simulink model "Quadrotor_Observer"  (Simulink 7.7)
settings: Solver=ode45  StartTime=0.0  StopTime=2  RelTol=1e-3
undefined symbols (not defined in the file or in its folder): quad
settings Model: Creator=Alexey  LastModifiedBy=Alexey

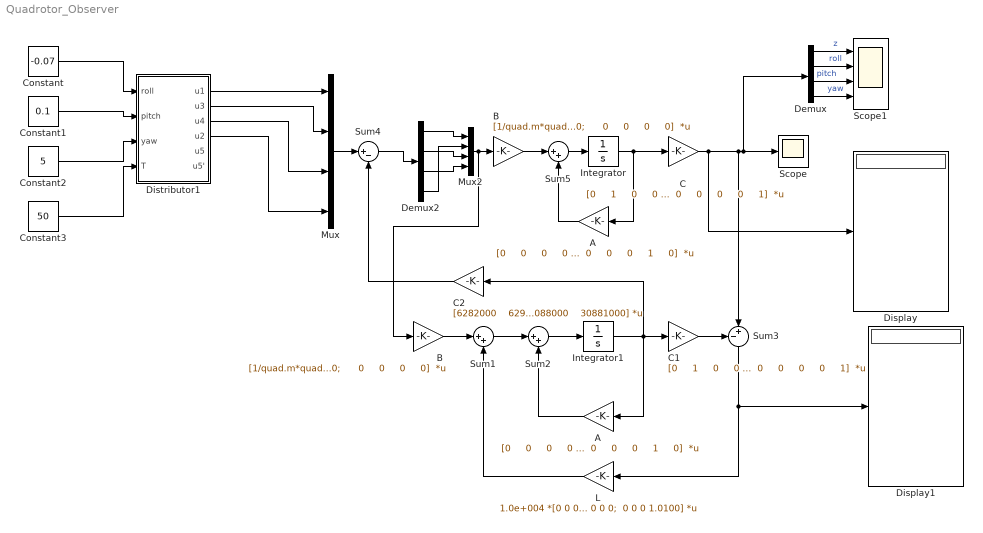
== system Quadrotor_Observer ==
  A : Gain  Gain=|  Multiplication=Matrix(K*u)
      | [0     0     0     0     0     0     0     0;
      |      1     0     0     0     0     0     0     0;
      |      0     0     0     0     0     0     0     0;
      |      0     0     1     0     0     0     0     0;
      |      0     0     0     0     0     0     0     0;
      |      0     0     0     0     1     0     0     0;
      |      0     0     0     0     0     0     0     0;
      |      0     0     0     0     0     0     1     0]
  "A " : Gain  Gain=|  Multiplication=Matrix(K*u)
      | [0     0     0     0     0     0     0     0;
      |      1     0     0     0     0     0     0     0;
      |      0     0     0     0     0     0     0     0;
      |      0     0     1     0     0     0     0     0;
      |      0     0     0     0     0     0     0     0;
      |      0     0     0     0     1     0     0     0;
      |      0     0     0     0     0     0     0     0;
      |      0     0     0     0     0     0     1     0]
  B : Gain  Gain=|  Multiplication=Matrix(K*u)
      | [1/quad.m*quad.b     0     0     0;
      |      0     0     0     0;
      |      0     0     1/quad.Ixx*quad.b*quad.l     0;
      |      0     0     0     0;
      |      0     0     0     1/quad.Iyy*quad.b*quad.l;
      |      0     0     0     0;
      |      0     1/quad.Izz*quad.k     0     0;
      |      0     0     0     0]
  "B " : Gain  Gain=|  Multiplication=Matrix(K*u)
      | [1/quad.m*quad.b     0     0     0;
      |      0     0     0     0;
      |      0     0     1/quad.Ixx*quad.b*quad.l     0;
      |      0     0     0     0;
      |      0     0     0     1/quad.Iyy*quad.b*quad.l;
      |      0     0     0     0;
      |      0     1/quad.Izz*quad.k*quad.r     0     0;
      |      0     0     0     0]
  C : Gain  Gain=|  Multiplication=Matrix(K*u)
      | [0     1     0     0     0     0     0     0;
      |      0     0     0     1     0     0     0     0;
      |      0     0     0     0     0     1     0     0;
      |      0     0     0     0     0     0     0     1]
  C1 : Gain  Gain=|  Multiplication=Matrix(K*u)
      | [0     1     0     0     0     0     0     0;
      |      0     0     0     1     0     0     0     0;
      |      0     0     0     0     0     1     0     0;
      |      0     0     0     0     0     0     0     1]
  C2 : Gain  Gain=|  Multiplication=Matrix(K*u)
      | [6282000    62976000 0 0 0 0 0 0;
      |       0 0 889700     2896900 0 0 0 0;
      |       0 0 0 0 889700     2896900 0 0;
      |     0 0 0 0 0 0 63088000    30881000]
  Constant : Constant  Value=-0.07
  Constant1 : Constant  Value=0.1
  Constant2 : Constant  Value=5
  Constant3 : Constant  Value=50
  Demux : Demux
  Demux2 : Demux
  Display : Display
  Display1 : Display
  Distributor1 : Subsystem
  Integrator : Integrator
  Integrator1 : Integrator
  L : Gain  Gain=|  Multiplication=Matrix(K*u)
      | 1.0e+004 *[0 0 0 0; 
      | 1.0100 0 0 0; 
      | 0 0 0 0; 
      | 0 1.0100 0 0; 
      | 0 0 0 0; 
      | 0 0 1.0100 0; 
      | 0 0 0 0; 
      | 0 0 0 1.0100]
  Mux : Mux
  Mux2 : Mux
  Scope : Scope
      settings: TimeRange=1
  Scope1 : Scope  NumInputPorts=4
      settings: TimeRange=1  YMin=0.99675~5~-8.4~0.7  YMax=0.9985~7~-7~0.78
  Sum1 : Sum  Inputs=|++
  Sum2 : Sum  Inputs=|++
  Sum3 : Sum  Inputs=-+|
  Sum4 : Sum  Inputs=|+-
  Sum5 : Sum  Inputs=|++
  wires:
  Sum4/1 -> Demux2/1
  B/1 -> Sum5/1
  Sum5/1 -> Integrator/1
  Integrator/1 -> C/1, "A "/1
  C/1 -> Sum3/2, Scope/1, Demux/1, Display/1
  "A "/1 -> Sum5/2
  Sum1/1 -> Sum2/1
  Sum2/1 -> Integrator1/1
  Integrator1/1 -> C1/1, A/1, C2/1
  C1/1 -> Sum3/1
  A/1 -> Sum2/2
  Sum3/1 -> Display1/1, L/1
  L/1 -> Sum1/2
  C2/1 -> Sum4/2
  "B "/1 -> Sum1/1
  Mux/1 -> Sum4/1
  Constant/1 -> Distributor1/1(roll)
  Constant1/1 -> Distributor1/2(pitch)
  Constant3/1 -> Distributor1/4(T)
  Constant2/1 -> Distributor1/3(yaw)
  Distributor1/1("u1 ") -> Mux/1
  Distributor1/4("u2 ") -> Mux/4
  Distributor1/2("u3 ") -> Mux/2
  Distributor1/3("u4 ") -> Mux/3
  Demux/1 -> Scope1/1  "z"
  Demux/2 -> Scope1/2  "roll"
  Demux/3 -> Scope1/3  "pitch"
  Demux/4 -> Scope1/4  "yaw"
  Demux2/1 -> Mux2/1
  Demux2/4 -> Mux2/2
  Demux2/2 -> Mux2/3
  Demux2/3 -> Mux2/4
  Mux2/1 -> B/1, "B "/1

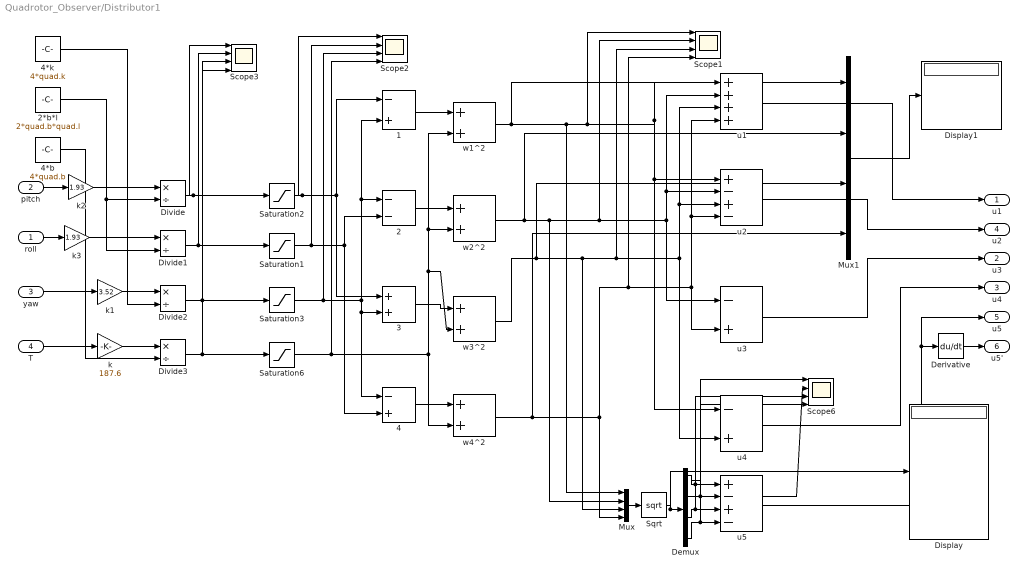
== system Quadrotor_Observer/Distributor1 ==
  roll : Inport
  pitch : Inport  Port=2
  yaw : Inport  Port=3
  T : Inport  Port=4
  1 : Sum  Inputs=-+
  2 : Sum  Inputs=--
  2*b*l : Constant  Value=2*quad.b*quad.l
  3 : Sum
  4 : Sum  Inputs=-+
  4*b : Constant  Value=4*quad.b
  4*k : Constant  Value=4*quad.k
  Demux : Demux
  Derivative : Derivative
  Display : Display
  Display1 : Display
  Divide{,1..3} (4 alike) : Product  Inputs=*/
  Mux : Mux
  Mux1 : Mux
  Saturation1 : Saturate  UpperLimit=287850  LowerLimit=-287850
  Saturation2 : Saturate  UpperLimit=287850  LowerLimit=-287850
  Saturation3 : Saturate  UpperLimit=9000000000  LowerLimit=-9000000000  LinearizeAsGain=off
  Saturation6 : Saturate  UpperLimit=1574000000  LowerLimit=15740000
  Scope{1..3,6} (4 alike) : Scope  NumInputPorts=4
      Scope1 settings: TimeRange=1  YMin=-5~-5~-5~-5  YMax=5~5~5~5  SaveName=ScopeData2
      Scope2 settings: TimeRange=1  YMin=-5~-5~-5~-5  YMax=5~5~5~5  SaveName=ScopeData4
      Scope3 settings: TimeRange=1  YMin=-5~-5~-5~-5  YMax=5~5~5~5  SaveName=ScopeData5
      Scope6 settings: TimeRange=1  YMin=-5~-5~-5~-5  YMax=5~5~5~5  SaveName=ScopeData6
  Sqrt : Sqrt  SaturateOnIntegerOverflow=on
  k : Gain  Gain=187.6
  k1 : Gain  Gain=3.52
  k2 : Gain  Gain=1.93
  k3 : Gain  Gain=1.93
  u1 : Sum  Inputs=++++
  u2 : Sum  Inputs=+-+-
  u3 : Sum  Inputs=-+
  u4 : Sum  Inputs=-+
  u5 : Sum  Inputs=+-+-
  w1^2 : Sum
  w2^2 : Sum
  w3^2 : Sum
  w4^2 : Sum
  "u1 " : Outport
  "u3 " : Outport  Port=2
  "u4 " : Outport  Port=3
  "u2 " : Outport  Port=4
  "u5 " : Outport  Port=5
  u5' : Outport  Port=6
  wires:
  4*k/1 -> Divide2/2
  Divide1/1 -> Scope3/2, Saturation1/1
  Divide2/1 -> Scope3/3, Saturation3/1
  Divide/1 -> Scope3/1, Saturation2/1
  4*b/1 -> Divide3/2
  yaw/1 -> k1/1
  2*b*l/1 -> Divide/2, Divide1/2
  roll/1 -> k3/1
  pitch/1 -> k2/1
  w1^2/1 -> Mux/1, u1/1, u2/1, u4/1, Scope1/1, Mux1/1
  w2^2/1 -> Mux/2, u1/2, u2/2, u3/1, Scope1/2, Mux1/2
  w3^2/1 -> Mux/3, u1/3, u2/3, u4/2, Scope1/3, Mux1/3
  w4^2/1 -> Mux/4, u1/4, u2/4, u3/2, Scope1/4, Mux1/4
  Divide3/1 -> Scope3/4, Saturation6/1
  T/1 -> k/1
  u1/1 -> "u1 "/1
  u2/1 -> "u2 "/1
  u3/1 -> "u3 "/1
  u4/1 -> "u4 "/1
  Mux/1 -> Sqrt/1
  Sqrt/1 -> Demux/1, Display/1
  Demux/1 -> u5/1, Scope6/1
  Demux/3 -> u5/3, Scope6/3
  Demux/2 -> u5/2, Scope6/2
  Demux/4 -> u5/4, Scope6/4
  u5/1 -> Derivative/1, "u5 "/1
  Derivative/1 -> u5'/1
  1/1 -> w1^2/1
  2/1 -> w2^2/1
  3/1 -> w3^2/1
  4/1 -> w4^2/1
  Saturation6/1 -> w1^2/2, w2^2/2, w3^2/2, w4^2/2, Scope2/4
  Mux1/1 -> Display1/1
  Saturation2/1 -> 1/1, 3/1, Scope2/1
  Saturation1/1 -> 2/2, 4/2, Scope2/2
  Saturation3/1 -> 3/2, 4/1, 1/2, 2/1, Scope2/3
  k2/1 -> Divide/1
  k3/1 -> Divide1/1
  k1/1 -> Divide2/1
  k/1 -> Divide3/1
